simulink model "controllerInputModel"  (R2025a)
settings: Solver=VariableStepAuto  StartTime=0.0  StopTime=inf  RelTol=1e-3
undefined symbols (not defined in the file): axes, buttons
libraries: ros2lib x2, sl3dlib x1
settings Model: Creator=hazem-m-abdelaziz  LastModifiedBy=hazem-m-abdelaziz
settings DebuggingCC: InheritedTsInSrcMsg=none

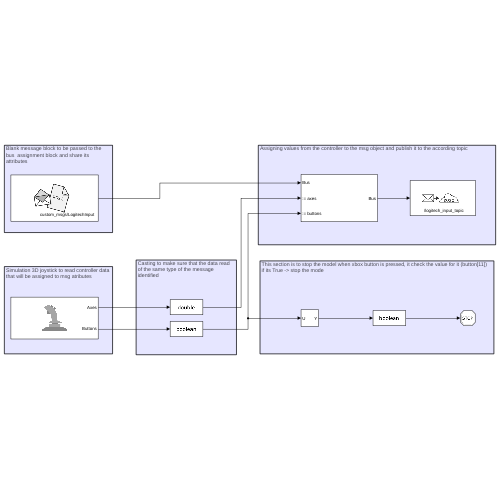
[thumbnail: Simulink's stored preview of the top-level diagram]
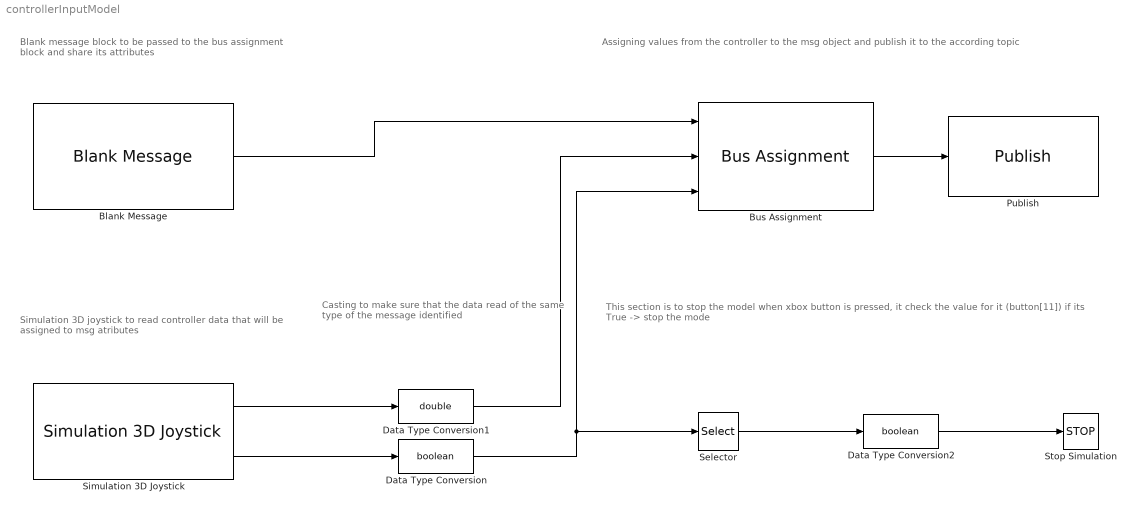
== system controllerInputModel ==
  note: Casting to make sure that the data read
      | of the same type of the message
      | identified
  note: Assigning values from the controller to the msg object and publish it to the according topic
  note: This section is to stop the model when xbox button is pressed, it check the value for it (button[11])
      | if its True -> stop the mode
  note: Simulation 3D joystick to read controller data
      | that will be assigned to msg atributes
  note: Blank message block to be passed to the
      | bus  assignment block and share its
      | attributes
  Blank Message : ros2lib/Blank Message  messageClass=Message  entityType=custom_msgs/LogitechInput  messageType=custom_msgs/LogitechInput  SampleTime=inf
  Bus Assignment : BusAssignment  AssignedSignals=axes,buttons
  Data Type Conversion : DataTypeConversion  OutDataTypeStr=boolean  SaturateOnIntegerOverflow=off  RndMeth=Floor
  Data Type Conversion1 : DataTypeConversion  OutDataTypeStr=double  SaturateOnIntegerOverflow=off  RndMeth=Floor
  Data Type Conversion2 : DataTypeConversion  OutDataTypeStr=boolean  SaturateOnIntegerOverflow=off  RndMeth=Floor
  Publish : ros2lib/Publish  topicSource=Specify your own  topic=/logitech_input_topic  messageType=custom_msgs/LogitechInput  QOSHistory=Keep last  QOSDepth=10  QOSReliability=Reliable  QOSDurability=Volatile  QOSDeadline=Inf  QOSLifespan=Inf  QOSLiveliness=Automatic  QOSLeaseDuration=Inf  QOSAvoidROSNamespaceConventions=off
  Selector : Selector  InputPortWidth=13  IndexOptions=Index vector (dialog)  Indices=11  OutputSizes=1
  Simulation 3D Joystick : sl3dlib/Simulation 3D/Hardware Interface/Simulation 3D Joystick  joyid=1  adjustports=on  forcefeed=off
  Stop Simulation : Stop
  wires:
  Blank Message/1 -> Bus Assignment/1
  Bus Assignment/1 -> Publish/1
  Simulation 3D Joystick/2 -> Data Type Conversion/1
  Simulation 3D Joystick/1 -> Data Type Conversion1/1
  Data Type Conversion1/1 -> Bus Assignment/2
  Data Type Conversion/1 -> Bus Assignment/3, Selector/1
  Selector/1 -> Data Type Conversion2/1
  Data Type Conversion2/1 -> Stop Simulation/1
